simulink model "Lab7a"  (Simulink 7.4)
settings: Solver=ode23tb  StartTime=0.0  StopTime=8  MaxStep=100e-6  RelTol=1e-3
libraries: powerlib x4, powerlib_extras x2
settings Model: Creator=msse9  LastModifiedBy=msse9

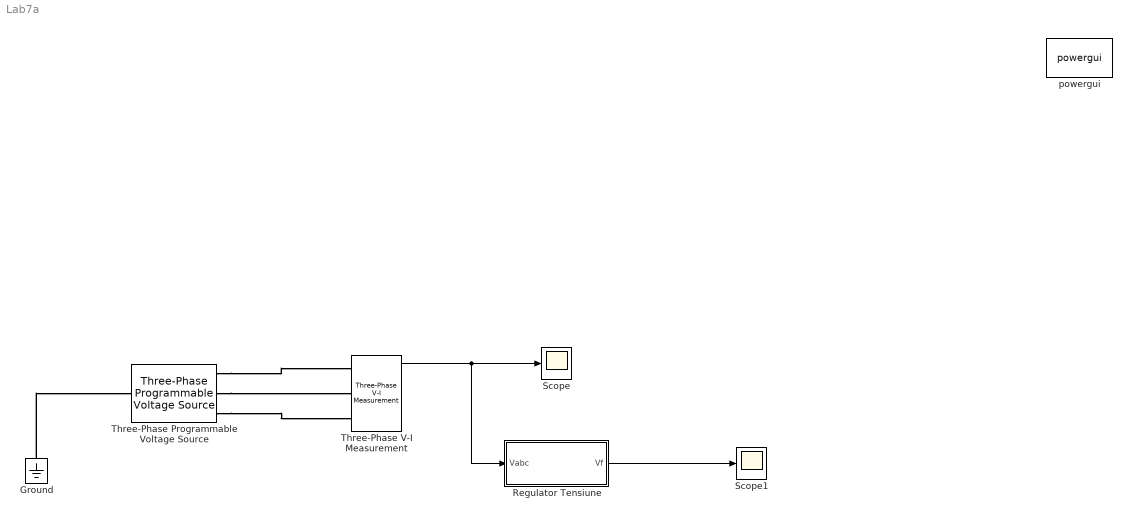
== system Lab7a ==
  Ground : powerlib/Elements/Ground  DialogController=POWERSYS.PowerSysDialog  PhysicalDomain=powersysdomain  SubClassName=unknown  LeftPortType=p1  RightPortType=p1  LConnTagsString=a
  Regulator Tensiune : Subsystem
  Scope : Scope
  Scope1 : Scope
      settings: YMin=-1  YMax=11
  Three-Phase Programmable Voltage Source : powerlib/Electrical Sources/Three-Phase Programmable Voltage Source  DialogController=POWERSYS.PowerSysDialog  SystemSampleTime=-1  PositiveSequence="[400  0 50]"  VariationEntity=Amplitude  VariationType=Step  VariationStep=-0.1  VariationRate=10  VariationMagnitude=0.3  VariationFrequency=2  VariationTiming=[2 10]  VariationPhaseA=off  Amplitudes=[1 0.8 1.2 1.0]  TimeValues=[0 0.1 0.15 0.2]  HarmonicGeneration=off  HarmonicA=[3 0.2 -25 0]  HarmonicB=[2 0.15 35 2]  Timing="[0.05  3]"
  Three-Phase V-I Measurement : powerlib/Measurements/Three-Phase V-I Measurement  DialogController=POWERSYS.PowerSysDialog  SystemSampleTime=-1  VoltageMeasurement=phase-to-ground  SetLabelV=off  LabelV=Vabc  Vpu=off  CurrentMeasurement=yes  SetLabelI=off  LabelI=Iabc  Ipu=off  Pbase=100e6  Vbase=500e3  OutputType=Complex  PhasorSimulation=off  PSBequivalent=0
  powergui : powerlib/powergui  Priority=1  SystemSampleTime=-1  SimulationMode=Continuous  SampleTime=50e-6  frequency=60  SPID=off  DisableSnubberDevices=off  DisableRonSwitches=off  DisableVfSwitches=off  SwTol=0  Interpol=off  frequencyindice=50  echomessages=off  HookPort=off  DisplayEquations=off  FunctionMessages=off  EnableUseOfTLC=off  x0status=blocks  RestoreLinks=warning  Frange=[0:2:500]  Ylog=off  Xlog=on  ShowGrid=off  save=off  variable=ZData  ZoomFFT=on  StartTime=0.0  cycles=1  DisplayStyle=1  fundamental=60  FreqAxis=off  MaxFrequency=1000  frequencyindicesteady=1  RmsSteady=1  display=off  Ts=0  methode=off
  wires:
  Three-Phase V-I Measurement/1 -> Scope/1, Regulator Tensiune/1(Vabc)
  Regulator Tensiune/1(Vf) -> Scope1/1
  connections:
  Ground/LConn1 -- Three-Phase Programmable Voltage Source/LConn1
  Three-Phase Programmable Voltage Source/RConn1 -- Three-Phase V-I Measurement/LConn1
  Three-Phase Programmable Voltage Source/RConn2 -- Three-Phase V-I Measurement/LConn2
  Three-Phase Programmable Voltage Source/RConn3 -- Three-Phase V-I Measurement/LConn3

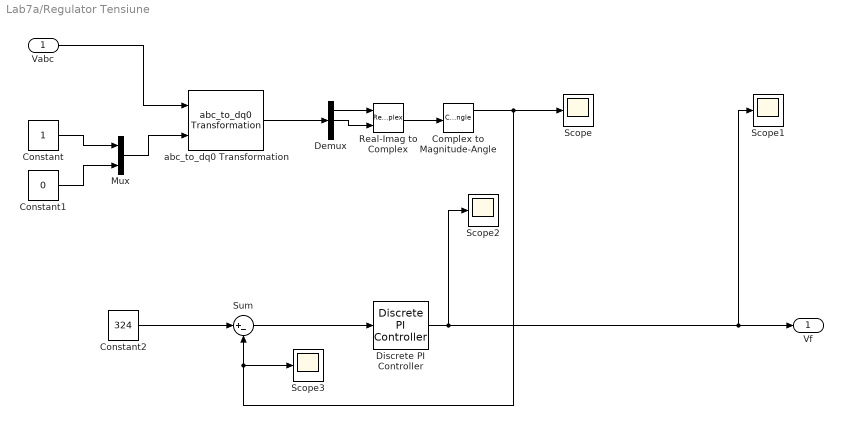
== system Lab7a/Regulator Tensiune ==
  Vabc : Inport  OutDataType=fixdt(1, 16)  OutScaling=2^0
  Complex to Magnitude-Angle : ComplexToMagnitudeAngle
  Constant : Constant  OutDataType=fixdt(1, 16)  OutScaling=2^0
  Constant1 : Constant  Value=0  OutDataType=fixdt(1, 16)  OutScaling=2^0
  Constant2 : Constant  Value=324  OutDataType=fixdt(1, 16)  OutScaling=2^0
  Demux : Demux  Outputs=3
  Discrete PI Controller : powerlib_extras/Discrete  Control Blocks/Discrete PI Controller  DialogController=POWERSYS.PowerSysDialog  SystemSampleTime=-1  Kp=0.01  Ki=0.04  Par_Limits=[10 0]  Init=0  Ts=1e-3
  Mux : Mux  Inputs=2
  Real-Imag to Complex : RealImagToComplex
  Scope{,1..3} (4 alike) : Scope
      Scope settings: SaveName=ScopeData2
      Scope1 settings: SaveName=ScopeData3
      Scope2 settings: SaveName=ScopeData4
      Scope3 settings: SaveName=ScopeData5
  Sum : Sum  Inputs=|+-  OutDataType=fixdt(1, 16)  OutScaling=2^0
  abc_to_dq0 Transformation : powerlib_extras/Measurements/abc_to_dq0 Transformation  DialogController=POWERSYS.PowerSysDialog  SystemSampleTime=-1
  Vf : Outport  OutDataType=fixdt(1, 16)  OutScaling=2^0
  wires:
  Vabc/1 -> abc_to_dq0 Transformation/1
  Constant/1 -> Mux/1
  Constant1/1 -> Mux/2
  Mux/1 -> abc_to_dq0 Transformation/2
  abc_to_dq0 Transformation/1 -> Demux/1
  Demux/1 -> Real-Imag to Complex/1
  Demux/2 -> Real-Imag to Complex/2
  Real-Imag to Complex/1 -> Complex to Magnitude-Angle/1
  Constant2/1 -> Sum/1
  Sum/1 -> Discrete PI Controller/1
  Discrete PI Controller/1 -> Vf/1, Scope1/1, Scope2/1
  Complex to Magnitude-Angle/1 -> Scope/1, Sum/2, Scope3/1
